simulink model "labgantryint"  (Simulink 6.3)
settings: Solver=ode1  SolverMode=SingleTasking  StartTime=0.0  StopTime=inf  FixedStep=0.001  RelTol=1e-3
values from neighbouring files (symbols this model uses):
  K = place( A, B, cl_poles )    [d_ip02_spg_pp.m]    (also in setup_lab_ip02_spg.m = [ 0 0 0 0 ])
  wcf = 2 * pi * 10    (= 62.8318530718)    [setup_lab_ip02_spg.m]
  X_LIM_ENABLE = 1    [setup_lab_ip02_spg.m]
  X_MAX = 0.25    [setup_lab_ip02_spg.m]
  X_MIN = - X_MAX    (= -0.25)    [setup_lab_ip02_spg.m]
  zetaf = 0.9    [setup_lab_ip02_spg.m]
libraries: qctools x5, simulink x2
settings Model: LastModifiedBy=localadmin  ExtModeArmWhenConnect=off  BufferReuse=off  StrictBusMsg=None
settings ConfigSet: SimulationMode=external
settings OptimizationCC: BooleanDataType=off  InlineInvariantSignals=on  OptimizeBlockIOStorage=off  BufferReuse=off  ExpressionFolding=off  LocalBlockOutputs=off
settings RTWCC: SystemTargetFile=wincon.tlc  MakeCommand=make_wc  TemplateMakefile=wc_default_tmf  Description=WinCon Target  ProcessScript=wincon_make_rtw_hook
settings STFCustomTargetCC: TargetFcnLib=ansi_tfl_tmw.mat  GenFloatMathFcnCalls=ANSI_C  ModelReferenceCompliant=off  SystemTargetFile=wincon.tlc
settings GRTTargetCC: ModelReferenceCompliant=off  MatFileLogging=off  ExtMode=on  ExtModeTransport=2  ExtModeMexFile=wc_comm
settings CustomProperty: Value=on

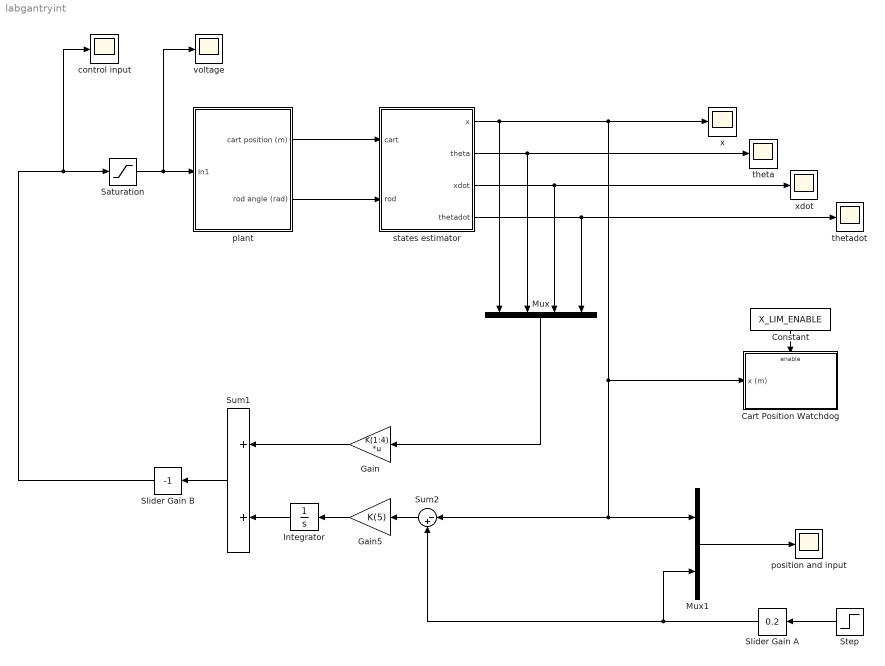
== system labgantryint ==
  Cart Position Watchdog : Subsystem  TreatAsAtomicUnit=on
  Constant : Constant  Orientation=down  Value=X_LIM_ENABLE
  Gain : Gain  Orientation=left  Gain=K(1:4)  Multiplication=Matrix(K*u)
  Gain5 : Gain  Orientation=left  Gain=K(5)
  Integrator : Integrator  Orientation=left
  Mux : Mux  Orientation=down
  Mux1 : Mux  Inputs=2
  Saturation : Saturate  UpperLimit=6  LowerLimit=-6
  Slider Gain A : simulink/Math Operations/Slider Gain  Orientation=left  low=-0.2  gain=0.2  high=0.2
  Slider Gain B : simulink/Math Operations/Slider Gain  Orientation=left  low=-1  gain=-1  high=1
  Step : Step  Orientation=left  SampleTime=0
  Sum1 : Sum  Orientation=left
  Sum2 : Sum  Orientation=left  Inputs=|-+
  control input : Scope
      settings: SaveName=ScopeData3
  plant : Subsystem
  position and input : Scope
      settings: SaveName=ScopeData6
  states estimator : Subsystem
  theta : Scope
  thetadot : Scope
      settings: SaveName=ScopeData2
  voltage : Scope
      settings: SaveName=ScopeData5
  x : Scope
      settings: SaveName=ScopeData4
  xdot : Scope
  wires:
  Slider Gain B/1 -> Saturation/1, control input/1
  plant/1(cart position (m)) -> states estimator/1(cart)
  plant/2(rod angle (rad)) -> states estimator/2(rod)
  states estimator/1(x) -> x/1, Sum2/1, Mux1/1, Cart Position Watchdog/1(x (m)), Mux/1
  states estimator/2(theta) -> theta/1, Mux/2
  states estimator/3(xdot) -> xdot/1, Mux/3
  states estimator/4(thetadot) -> thetadot/1, Mux/4
  Sum1/1 -> Slider Gain B/1
  Saturation/1 -> plant/1(In1), voltage/1
  Sum2/1 -> Gain5/1
  Gain5/1 -> Integrator/1
  Integrator/1 -> Sum1/2
  Slider Gain A/1 -> Sum2/2, Mux1/2
  Constant/1 -> Cart Position Watchdog/Enable
  Mux/1 -> Gain/1
  Gain/1 -> Sum1/1
  Mux1/1 -> position and input/1
  Step/1 -> Slider Gain A/1

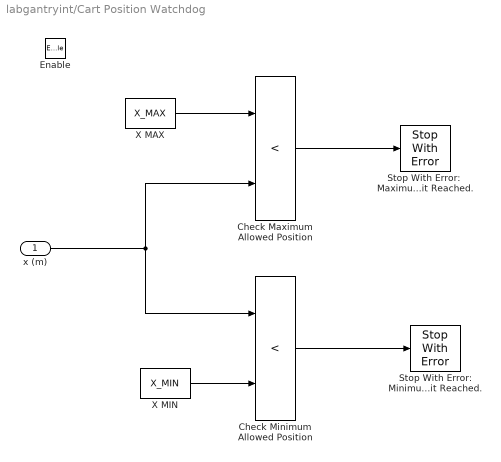
== system labgantryint/Cart Position Watchdog ==
  x (m) : Inport
  Enable : EnablePort
  Check Maximum Allowed Position : RelationalOperator  Operator=<  InputSameDT=on
  Check Minimum Allowed Position : RelationalOperator  Operator=<  InputSameDT=on
  Stop With Error: Minimum Limit Reached. : qctools/Extra Sinks/Stop With Error  errMsg=Minimum Position Limit reached.
  Stop With Error:  Maximum Limit Reached. : qctools/Extra Sinks/Stop With Error  errMsg=Maximum Position Limit reached.
  X MAX : Constant  Value=X_MAX
  X MIN : Constant  Value=X_MIN
  wires:
  Check Maximum Allowed Position/1 -> Stop With Error:  Maximum Limit Reached./1
  x (m)/1 -> Check Minimum Allowed Position/1, Check Maximum Allowed Position/2
  X MIN/1 -> Check Minimum Allowed Position/2
  Check Minimum Allowed Position/1 -> Stop With Error: Minimum Limit Reached./1
  X MAX/1 -> Check Maximum Allowed Position/1

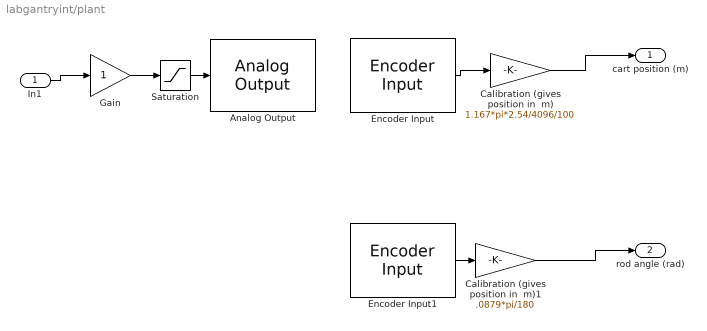
== system labgantryint/plant ==
  In1 : Inport
  Analog Output : qctools/Quanser Q4 Series/Analog Output  boardNumber=0  channels=0  modesVect=0  rangesVect=10  initialVect=0  finalVect=0  sampleTime=-1  inputVolts=on  simulationOutput=off
  Calibration (gives position in  m) : Gain  Gain=1.167*pi*2.54/4096/100  SaturateOnIntegerOverflow=on
  Calibration (gives position in  m)1 : Gain  Gain=.0879*pi/180  SaturateOnIntegerOverflow=on
  Encoder Input : qctools/Quanser Q4 Series/Encoder Input  boardNumber=0  channels=0  initial=0  preserveCounts=off  sampleTime=default_sample_time  quadratureStr=4X  modeStr=Normal  flagString=FLG1 is IDX and FLG2 is E  prescale=1  frequency=16666666.6667  use33MHzClock=off  bcd=off  enableIndex=on  synchronousIndex=on  indexPolarity=on  reloadOnIndex=off  simulationInput=off
  Encoder Input1 : qctools/Quanser Q4 Series/Encoder Input  boardNumber=0  channels=1  initial=0  preserveCounts=off  sampleTime=default_sample_time  quadratureStr=4X  modeStr=Normal  flagString=FLG1 is IDX and FLG2 is E  prescale=1  frequency=16666666.6667  use33MHzClock=off  bcd=off  enableIndex=on  synchronousIndex=on  indexPolarity=on  reloadOnIndex=off  simulationInput=off
  Gain : Gain  SaturateOnIntegerOverflow=on
  Saturation : Saturate  UpperLimit=6  LowerLimit=-6
  cart position (m) : Outport
  rod angle (rad) : Outport  Port=2
  wires:
  Encoder Input/1 -> Calibration (gives position in  m)/1
  Calibration (gives position in  m)/1 -> cart position (m)/1
  Calibration (gives position in  m)1/1 -> rod angle (rad)/1
  Encoder Input1/1 -> Calibration (gives position in  m)1/1
  Saturation/1 -> Analog Output/1
  In1/1 -> Gain/1
  Gain/1 -> Saturation/1

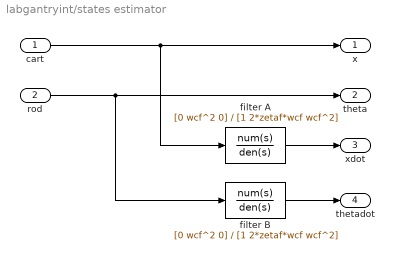
== system labgantryint/states estimator ==
  cart : Inport
  rod : Inport  Port=2
  filter A : TransferFcn  Numerator=[0 wcf^2 0]  Denominator=[1 2*zetaf*wcf wcf^2]
  filter B : TransferFcn  Numerator=[0 wcf^2 0]  Denominator=[1 2*zetaf*wcf wcf^2]
  x : Outport
  theta : Outport  Port=2
  xdot : Outport  Port=3
  thetadot : Outport  Port=4
  wires:
  cart/1 -> x/1, filter A/1
  rod/1 -> theta/1, filter B/1
  filter A/1 -> xdot/1
  filter B/1 -> thetadot/1
